simulink model "State_Flowc"  (R2017a)
settings: Solver=FixedStepDiscrete  StartTime=0.0  StopTime=inf  FixedStep=0.001  RelTol=1e-3  EnableMultiTasking=on
libraries: xpcethercatlib x31, simulink x4, simulink_extras x4, commutil2 x2
(part 1 of 2)
settings Model: xpc_rtwmakecfg_data=_xpcethercatlib_  SimulationMode=external  Creator=simoc  LastModifiedBy=Danie
settings SolverCC: EnableConcurrentExecution=on  ConcurrentTasks=on  AutoInsertRateTranBlk=on
settings DataIOCC: SaveFormat=StructureWithTime
settings OptimizationCC: BlockReduction=off  OptimizeBlockIOStorage=off  BufferReuse=off  GlobalBufferReuse=off  ExpressionFolding=off  LocalBlockOutputs=off
settings HardwareCC: ProdBitPerPointer=32  ProdBitPerSizeT=32  ProdBitPerPtrDiffT=32  ProdLargestAtomicFloat=None  ProdWordSize=32  ProdLongLongMode=on  ProdHWDeviceType=Generic->32-bit x86 compatible
settings RTWCC: SystemTargetFile=slrt.tlc  TemplateMakefile=slrt_default_tmf  Description=Simulink Real-Time  RTWCompilerOptimization=on
settings SimulinkRealTimeCC: xPCConcurrentTasks=on

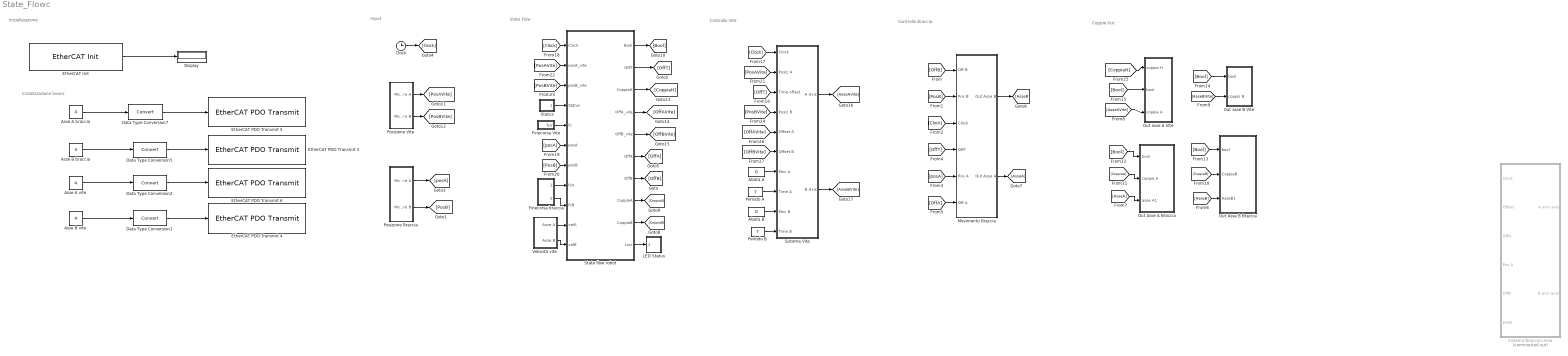
== system State_Flowc ==
  note: Input
  note: State Flow
  note: Coppie Out
  note: Controllo Braccia
  note: Controllo Vite
  note: Inizializzazione
  note: Inizializzazione lavoro
  Alzata A : Constant  Value=0
  "Alzata B " : Constant  Value=0
  Asse A braccia : Constant  Value=4
  Asse A vite : Constant  Value=4
  Asse B braccia : Constant  Value=4
  Asse B vite : Constant  Value=4
  Clock : Clock
  Data Type Conversion{1..2,5,7} (4 alike) : DataTypeConversion
  Display : Display
  "EtherCAT Init " : xpcethercatlib/EtherCAT Init   Priority=0  config_file=C:\Users\Danie\Downloads\final_net.xml  device_id=0  pci_bus=4  pci_slot=1  dctuning=0  enaDebug=off  enaDC=on  errLink=off  masterDbg=off  stateChgDbg=off  baseClock=off  masterCfg=off  logFile='c:\dbglog.txt'  sample_time=0.001000  DCMode=1
      settings: SourceProductName=Simulink Real-Time  SourceProductBaseCode=XP
  EtherCAT PDO Transmit 3 : xpcethercatlib/EtherCAT PDO Transmit   Priority=3  sig_name=AZ2.Receive PDO 1.Axis A Modes of operation  sig_offset=264  sig_type=int8  type_size=8  sig_dim=1  device_id=0  sample_time=0.001000
      settings: SourceProductName=Simulink Real-Time  SourceProductBaseCode=XP
  EtherCAT PDO Transmit 4 : xpcethercatlib/EtherCAT PDO Transmit   Priority=3  sig_name=AZ2.Receive PDO 1.Axis A Modes of operation  sig_offset=264  sig_type=int8  type_size=8  sig_dim=1  device_id=0  sample_time=0.001000
      settings: SourceProductName=Simulink Real-Time  SourceProductBaseCode=XP
  EtherCAT PDO Transmit 5 : xpcethercatlib/EtherCAT PDO Transmit   Priority=3  sig_name=AZ2.Receive PDO 2.Axis B Modes of operation  sig_offset=288  sig_type=int8  type_size=8  sig_dim=1  device_id=0  sample_time=0.001000
      settings: SourceProductName=Simulink Real-Time  SourceProductBaseCode=XP
  EtherCAT PDO Transmit 6 : xpcethercatlib/EtherCAT PDO Transmit   Priority=3  sig_name=AZ2.Receive PDO 1.Axis A Modes of operation  sig_offset=264  sig_type=int8  type_size=8  sig_dim=1  device_id=0  sample_time=0.001000
      settings: SourceProductName=Simulink Real-Time  SourceProductBaseCode=XP
  Finecorsa Vite : Subsystem
  Finecorsa braccia : Subsystem
  LED Status : Subsystem
  Movimento Braccia : Subsystem
  Out Asse A Braccia : Subsystem
  Out Asse B Braccia : Subsystem
  Out asse A Vite : Subsystem
  Out asse B Vite : Subsystem
  Periodo A : Constant  Value=7
  Periodo B : Constant  Value=7
  "Posizione Braccia " : Subsystem
  Posizione Vite : Subsystem
  Sistema Braccia Linea : Subsystem  Commented=on
  Sistema Vite : Subsystem
  State flow robot : Stateflow chart  TreatAsAtomicUnit=on
  Status : Subsystem
  "Velocita vite " : Subsystem
  wires:
  "EtherCAT Init "/1 -> Display/1
  Data Type Conversion7/1 -> EtherCAT PDO Transmit 5/1
  Asse A braccia/1 -> Data Type Conversion7/1
  Data Type Conversion5/1 -> EtherCAT PDO Transmit 3/1
  Asse B braccia/1 -> Data Type Conversion5/1
  Clock/1 -> [Clock]
  State flow robot/1(Bool) -> [Bool]
  Data Type Conversion1/1 -> EtherCAT PDO Transmit 4/1
  Asse B vite/1 -> Data Type Conversion1/1
  Data Type Conversion2/1 -> EtherCAT PDO Transmit 6/1
  Asse A vite/1 -> Data Type Conversion2/1
  Posizione Vite/2(Motore B) -> [PosBVite]
  Status/1(Word) -> State flow robot/4(Status)
  State flow robot/2(OffT) -> [OffT]
  Alzata A/1 -> Sistema Vite/7(Mov A)
  Periodo A/1 -> Sistema Vite/8(Time A)
  "Alzata B "/1 -> Sistema Vite/9(Mov B)
  Periodo B/1 -> Sistema Vite/10(Time B)
  Finecorsa Vite/1(fcV) -> State flow robot/5(fc)
  Finecorsa braccia/1(Asse A) -> State flow robot/8(fcA)
  Finecorsa braccia/2(Asse B) -> State flow robot/9(fcB)
  "Posizione Braccia "/2(Motore B) -> [PosB]
  "Posizione Braccia "/1(Motore A) -> [posA]
  Posizione Vite/1(Motore A) -> [PosAVite]
  State flow robot/10(Luci) -> LED Status/1(Luci)
  "Velocita vite "/1(Asse A) -> State flow robot/10(velA)
  "Velocita vite "/2(Asse B) -> State flow robot/11(velB)
  State flow robot/7(OffB) -> [OffB]
  State flow robot/6(OffA) -> [OffA]
  [AsseB] -> Out Asse B Braccia/3(AsseB1)
  [AsseA] -> Out Asse A Braccia/3(asse A1)
  [CoppiaB] -> Out Asse B Braccia/2(CoppiaB)
  State flow robot/9(CoppiaB) -> [CoppiaB]
  State flow robot/8(CoppiaA) -> [CoppiaA]
  [CoppiaA] -> Out Asse A Braccia/2(coppia A)
  [Bool] -> Out Asse A Braccia/1(bool)
  [Bool] -> Out Asse B Braccia/1(bool)
  [Bool] -> Out asse B Vite/1(bool)
  [Bool] -> Out asse A Vite/2(bool)
  [OffT] -> Sistema Vite/3(Time offset)
  [Clock] -> Sistema Vite/1(Clock)
  [Clock] -> State flow robot/1(Clock)
  [posA] -> State flow robot/6(posA)
  [PosB] -> State flow robot/7(posB)
  [PosAVite] -> Sistema Vite/2(Posiz A)
  [PosAVite] -> State flow robot/2(posA_vite)
  [PosBVite] -> State flow robot/3(posB_vite)
  [PosBVite] -> Sistema Vite/4(Posiz B)
  State flow robot/3(CoppiaH) -> [CoppiaH]
  [CoppiaH] -> Out asse A Vite/1(coppia H)
  State flow robot/4(OffA_vite) -> [OffAVite]
  [OffAVite] -> Sistema Vite/5(Offset A)
  State flow robot/5(OffB_vite) -> [OffBVite]
  [OffBVite] -> Sistema Vite/6(Offset B)
  [OffB] -> Movimento Braccia/1(Off B)
  [PosB] -> Movimento Braccia/2(Pos B)
  [Clock] -> Movimento Braccia/3(Clock)
  [OffT] -> Movimento Braccia/4(OffT)
  [posA] -> Movimento Braccia/5(Pos A)
  [OffA] -> Movimento Braccia/6(Off A)
  Movimento Braccia/1(Out Asse B) -> [AsseB]
  Movimento Braccia/2(Out Asse A) -> [AsseA]
  Sistema Vite/1(A Axis) -> [AsseAVite]
  [AsseAVite] -> Out asse A Vite/3(coppia A)
  Sistema Vite/2(B Axis) -> [AsseBVite]
  [AsseBVite] -> Out asse B Vite/2(coppis B)

== system State_Flowc/Finecorsa Vite ==
  Data Type Conversion8 : DataTypeConversion
  EtherCAT PDO Receive16 : xpcethercatlib/EtherCAT PDO Receive  Priority=2  sig_name=AZ2.Transmit PDO 3.General purpose inputs  sig_offset=440  sig_type=uint16  type_size=16  sig_dim=1  device_id=0  sample_time=0.001000
      settings: SourceProductName=Simulink Real-Time  SourceProductBaseCode=XP
  Integer to Bit Converter : commutil2/Integer to Bit Converter  nbits=16  signedInputValues=Unsigned  bitOrder=LSB first  outDtype=Inherit via internal rule
  Selector : Selector  InputPortWidth=16  IndexOptions=Index vector (dialog)  Indices=15  OutputSizes=1
  fcV : Outport
  wires:
  EtherCAT PDO Receive16/1 -> Data Type Conversion8/1
  Selector/1 -> fcV/1
  Data Type Conversion8/1 -> Integer to Bit Converter/1
  Integer to Bit Converter/1 -> Selector/1

== system State_Flowc/Finecorsa braccia ==
  Data Type Conversion8 : DataTypeConversion
  EtherCAT PDO Receive16 : xpcethercatlib/EtherCAT PDO Receive  Priority=2  sig_name=AZ1.Transmit PDO 3.General purpose inputs  sig_offset=184  sig_type=uint16  type_size=16  sig_dim=1  device_id=0  sample_time=0.001000
      settings: SourceProductName=Simulink Real-Time  SourceProductBaseCode=XP
  Integer to Bit Converter : commutil2/Integer to Bit Converter  nbits=16  signedInputValues=Unsigned  bitOrder=LSB first  outDtype=Inherit via internal rule
  Selector : Selector  InputPortWidth=16  IndexOptions=Index vector (dialog)  Indices=8  OutputSizes=1
  Selector1 : Selector  InputPortWidth=16  IndexOptions=Index vector (dialog)  Indices=15  OutputSizes=1
  Asse A : Outport
  Asse B : Outport  Port=2
  wires:
  Data Type Conversion8/1 -> Integer to Bit Converter/1
  Integer to Bit Converter/1 -> Selector1/1, Selector/1
  EtherCAT PDO Receive16/1 -> Data Type Conversion8/1
  Selector1/1 -> Asse B/1
  Selector/1 -> Asse A/1

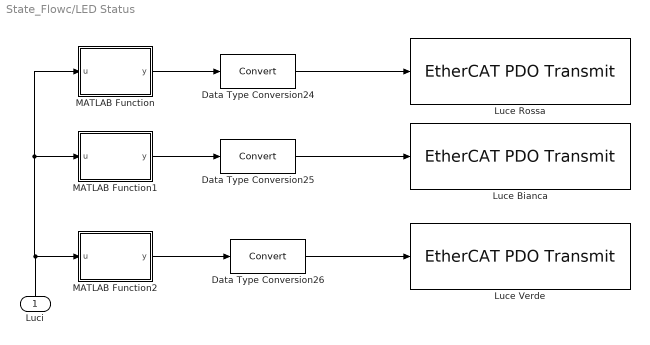
== system State_Flowc/LED Status ==
  Luci : Inport
  Data Type Conversion24 : DataTypeConversion
  Data Type Conversion25 : DataTypeConversion
  Data Type Conversion26 : DataTypeConversion
  Luce Bianca : xpcethercatlib/EtherCAT PDO Transmit   Priority=3  sig_name=Beckoff.Channel 6.Output  sig_offset=1  sig_type=boolean  type_size=1  sig_dim=1  device_id=0  sample_time=0.001000
      settings: SourceProductName=Simulink Real-Time  SourceProductBaseCode=XP
  "Luce Rossa " : xpcethercatlib/EtherCAT PDO Transmit   Priority=3  sig_name=Beckoff.Channel 8.Output  sig_offset=3  sig_type=boolean  type_size=1  sig_dim=1  device_id=0  sample_time=0.001000
      settings: SourceProductName=Simulink Real-Time  SourceProductBaseCode=XP
  Luce Verde : xpcethercatlib/EtherCAT PDO Transmit   Priority=3  sig_name=Beckoff.Channel 7.Output  sig_offset=2  sig_type=boolean  type_size=1  sig_dim=1  device_id=0  sample_time=0.001000
      settings: SourceProductName=Simulink Real-Time  SourceProductBaseCode=XP
  MATLAB Function : MATLAB Function  TreatAsAtomicUnit=on
  MATLAB Function1 : MATLAB Function  TreatAsAtomicUnit=on
  MATLAB Function2 : MATLAB Function  TreatAsAtomicUnit=on
  wires:
  MATLAB Function2/1(y) -> Data Type Conversion26/1
  MATLAB Function/1(y) -> Data Type Conversion24/1
  Data Type Conversion26/1 -> Luce Verde/1
  MATLAB Function1/1(y) -> Data Type Conversion25/1
  Data Type Conversion24/1 -> "Luce Rossa "/1
  Data Type Conversion25/1 -> Luce Bianca/1
  Luci/1 -> MATLAB Function/1(u), MATLAB Function1/1(u), MATLAB Function2/1(u)

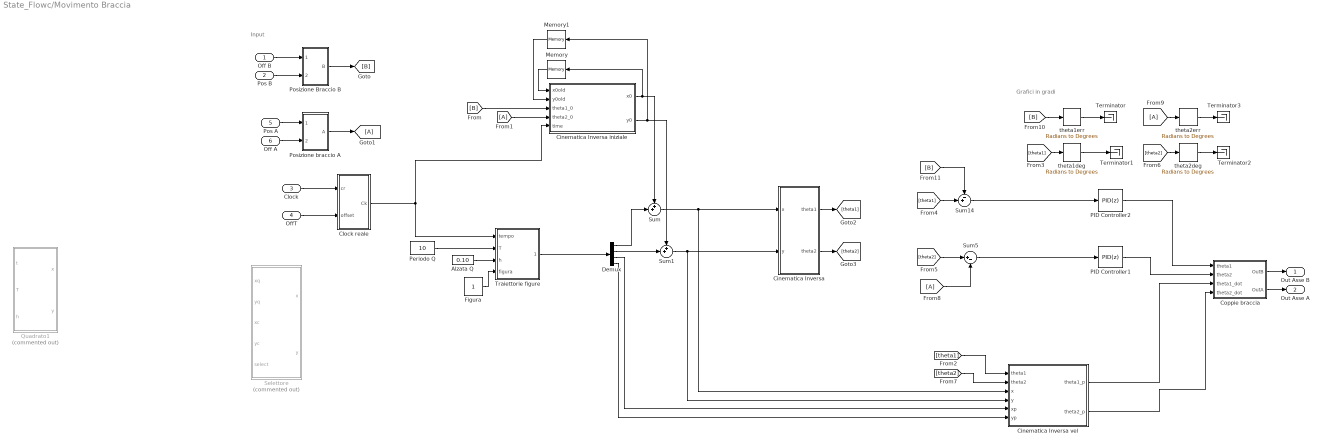
== system State_Flowc/Movimento Braccia ==
  note: Input
  note: Grafici in gradi
  Off B : Inport
  Pos B : Inport  Port=2
  Clock : Inport  Port=3
  OffT : Inport  Port=4
  Pos A : Inport  Port=5
  Off A : Inport  Port=6
  Alzata Q : Constant  Value=0.10
  Cinematica Inversa : MATLAB Function  TreatAsAtomicUnit=on
  Cinematica Inversa iniziale : MATLAB Function  TreatAsAtomicUnit=on
  Cinematica Inversa vel : MATLAB Function  TreatAsAtomicUnit=on
  Clock reale : Subsystem
  Coppie braccia : Subsystem
  Demux : Demux
  Figura : Constant
  Memory : Memory
  Memory1 : Memory
  PID Controller1 : simulink/Continuous/PID Controller  Controller=PID  TimeDomain=Discrete-time  SampleTime=-1  IntegratorMethod=Forward Euler  FilterMethod=Forward Euler  Form=Parallel  UseFilter=on  ControllerParametersSource=internal  P=3e+05  I=100  D=0  N=100  InitialConditionSource=internal  InitialConditionForIntegrator=0  InitialConditionForFilter=0  ExternalReset=none  LimitOutput=off  UpperSaturationLimit=inf  LowerSaturationLimit=-inf  LinearizeAsGain=on  AntiWindupMode=none  Kb=1  TrackingMode=off  Kt=1  PParamMin=[]  PParamMax=[]  IParamMin=[]  IParamMax=[]  DParamMin=[]  DParamMax=[]  NParamMin=[]  NParamMax=[]  KbParamMin=[]  KbParamMax=[]  KtParamMin=[]  KtParamMax=[]  POutMin=[]  POutMax=[]  IOutMin=[]  IOutMax=[]  DOutMin=[]  DOutMax=[]  NOutMin=[]  NOutMax=[]  KbOutMin=[]  KbOutMax=[]  KtOutMin=[]  KtOutMax=[]  IntegratorOutMin=[]  IntegratorOutMax=[]  FilterOutMin=[]  FilterOutMax=[]  SumOutMin=[]  SumOutMax=[]  SumI1OutMin=[]  SumI1OutMax=[]  SumI2OutMin=[]  SumI2OutMax=[]  SumI3OutMin=[]  SumI3OutMax=[]  SumDOutMin=[]  SumDOutMax=[]  SaturationOutMin=[]  SaturationOutMax=[]  IntegratorContinuousStateAttributes=''  IntegratorStateMustResolveToSignalObject=off  IntegratorRTWStateStorageClass=Auto  FilterContinuousStateAttributes=''  FilterStateMustResolveToSignalObject=off  FilterRTWStateStorageClass=Auto  DifferentiatorICPrevScaledInput=0  DifferentiatorOutMin=[]  DifferentiatorOutMax=[]  InitialConditionSetting=State (most efficient)
  PID Controller2 : simulink/Continuous/PID Controller  Controller=PID  TimeDomain=Discrete-time  SampleTime=-1  IntegratorMethod=Forward Euler  FilterMethod=Forward Euler  Form=Parallel  UseFilter=on  ControllerParametersSource=internal  P=3e+05  I=100  D=0  N=100  InitialConditionSource=internal  InitialConditionForIntegrator=0  InitialConditionForFilter=0  ExternalReset=none  LimitOutput=off  UpperSaturationLimit=inf  LowerSaturationLimit=-inf  LinearizeAsGain=on  AntiWindupMode=none  Kb=1  TrackingMode=off  Kt=1  PParamMin=[]  PParamMax=[]  IParamMin=[]  IParamMax=[]  DParamMin=[]  DParamMax=[]  NParamMin=[]  NParamMax=[]  KbParamMin=[]  KbParamMax=[]  KtParamMin=[]  KtParamMax=[]  POutMin=[]  POutMax=[]  IOutMin=[]  IOutMax=[]  DOutMin=[]  DOutMax=[]  NOutMin=[]  NOutMax=[]  KbOutMin=[]  KbOutMax=[]  KtOutMin=[]  KtOutMax=[]  IntegratorOutMin=[]  IntegratorOutMax=[]  FilterOutMin=[]  FilterOutMax=[]  SumOutMin=[]  SumOutMax=[]  SumI1OutMin=[]  SumI1OutMax=[]  SumI2OutMin=[]  SumI2OutMax=[]  SumI3OutMin=[]  SumI3OutMax=[]  SumDOutMin=[]  SumDOutMax=[]  SaturationOutMin=[]  SaturationOutMax=[]  IntegratorContinuousStateAttributes=''  IntegratorStateMustResolveToSignalObject=off  IntegratorRTWStateStorageClass=Auto  FilterContinuousStateAttributes=''  FilterStateMustResolveToSignalObject=off  FilterRTWStateStorageClass=Auto  DifferentiatorICPrevScaledInput=0  DifferentiatorOutMin=[]  DifferentiatorOutMax=[]  InitialConditionSetting=State (most efficient)
  Periodo Q : Constant  Value=10
  Posizione Braccio B : Subsystem
  Posizione braccio A : Subsystem
  Quadrato1 : MATLAB Function  Commented=on  TreatAsAtomicUnit=on
  Selettore : MATLAB Function  Commented=on  TreatAsAtomicUnit=on
  Sum : Sum  Inputs=++|
  Sum1 : Sum  Inputs=++|
  Sum14 : Sum  Inputs=-+|
  Sum5 : Sum  Inputs=|+-
  Terminator{,1..3} (4 alike) : Terminator
  Traiettorie figure : Subsystem
  theta1deg : simulink_extras/Transformations/Radians to Degrees
  theta1err : simulink_extras/Transformations/Radians to Degrees
  theta2deg : simulink_extras/Transformations/Radians to Degrees
  theta2err : simulink_extras/Transformations/Radians to Degrees
  Out Asse B : Outport
  Out Asse A : Outport  Port=2
  wires:
  Sum5/1 -> PID Controller1/1
  Cinematica Inversa iniziale/2(y0) -> Sum1/1, Memory1/1
  Sum/1 -> Cinematica Inversa vel/3(x), Cinematica Inversa/1(x)
  Sum1/1 -> Cinematica Inversa vel/4(y), Cinematica Inversa/2(y)
  Sum14/1 -> PID Controller2/1
  Clock/1 -> Clock reale/1(cr)
  OffT/1 -> Clock reale/2(offset)
  Clock reale/1(Ck) -> Cinematica Inversa iniziale/5(time), Traiettorie figure/1(tempo)
  Cinematica Inversa iniziale/1(x0) -> Sum/1, Memory/1
  Memory1/1 -> Cinematica Inversa iniziale/2(y0old)
  Memory/1 -> Cinematica Inversa iniziale/1(x0old)
  theta1deg/1 -> Terminator1/1
  theta1err/1 -> Terminator/1
  theta2deg/1 -> Terminator2/1
  theta2err/1 -> Terminator3/1
  Posizione Braccio B/1(B) -> [B]
  Off B/1 -> Posizione Braccio B/1(Off B)
  Pos B/1 -> Posizione Braccio B/2(Pos B)
  Posizione braccio A/1(A) -> [A]
  Pos A/1 -> Posizione braccio A/1(Pos A)
  Off A/1 -> Posizione braccio A/2(Off A)
  PID Controller2/1 -> Coppie braccia/1(theta1)
  PID Controller1/1 -> Coppie braccia/2(theta2)
  Cinematica Inversa vel/1(theta1_p) -> Coppie braccia/3(theta1_dot)
  Cinematica Inversa vel/2(theta2_p) -> Coppie braccia/4(theta2_dot)
  Coppie braccia/1(OutB) -> Out Asse B/1
  Coppie braccia/2(OutA) -> Out Asse A/1
  [B] -> Cinematica Inversa iniziale/3(theta1_0)
  [A] -> Cinematica Inversa iniziale/4(theta2_0)
  Demux/1 -> Sum/2
  Demux/2 -> Sum1/2
  Demux/3 -> Cinematica Inversa vel/5(xp)
  Demux/4 -> Cinematica Inversa vel/6(yp)
  Cinematica Inversa/1(theta1) -> [theta1]
  [theta1] -> Sum14/2
  [theta1] -> theta1deg/1
  [theta1] -> Cinematica Inversa vel/1(theta1)
  Cinematica Inversa/2(theta2) -> [theta2]
  [theta2] -> Sum5/1
  [theta2] -> theta2deg/1
  [theta2] -> Cinematica Inversa vel/2(theta2)
  [A] -> Sum5/2
  [A] -> theta2err/1
  [B] -> theta1err/1
  [B] -> Sum14/1
  Periodo Q/1 -> Traiettorie figure/2(T)
  Alzata Q/1 -> Traiettorie figure/3(h)
  Traiettorie figure/1(Parametri) -> Demux/1
  Figura/1 -> Traiettorie figure/4(figura)

== system State_Flowc/Out Asse A Braccia ==
  note: Invio motore asse A
  bool : Inport
  coppia A : Inport  Port=2
  asse A1 : Inport  Port=3
  Data Type Conversion3 : DataTypeConversion
  EtherCAT PDO Transmit 1 : xpcethercatlib/EtherCAT PDO Transmit   Priority=3  sig_name=AZ1.Receive PDO 1.Axis A Target Torque  sig_offset=16  sig_type=int16  type_size=16  sig_dim=1  device_id=0  sample_time=0.001000
      settings: SourceProductName=Simulink Real-Time  SourceProductBaseCode=XP
  Fungo : Subsystem
  Saturation : Saturate  UpperLimit=2500  LowerLimit=-2500
  Switch1 : Switch  Criteria=u2 > Threshold  Threshold=3
  wires:
  Data Type Conversion3/1 -> EtherCAT PDO Transmit 1/1
  bool/1 -> Switch1/2
  asse A1/1 -> Switch1/1
  coppia A/1 -> Switch1/3
  Switch1/1 -> Fungo/1(In1)
  Fungo/1(Out1) -> Saturation/1
  Saturation/1 -> Data Type Conversion3/1

== system State_Flowc/Out Asse B Braccia ==
  note: Invio motore Asse B
  bool : Inport
  CoppiaB : Inport  Port=2
  AsseB1 : Inport  Port=3
  Data Type Conversion4 : DataTypeConversion
  EtherCAT PDO Transmit 7 : xpcethercatlib/EtherCAT PDO Transmit   Priority=3  sig_name=AZ1.Receive PDO 2.Axis B Target Torque  sig_offset=40  sig_type=int16  type_size=16  sig_dim=1  device_id=0  sample_time=0.001000
      settings: SourceProductName=Simulink Real-Time  SourceProductBaseCode=XP
  Fungo : Subsystem
  Saturation : Saturate  UpperLimit=2500  LowerLimit=-2500
  Switch1 : Switch  Criteria=u2 > Threshold  Threshold=3
  wires:
  Data Type Conversion4/1 -> EtherCAT PDO Transmit 7/1
  AsseB1/1 -> Switch1/1
  Switch1/1 -> Fungo/1(In1)
  CoppiaB/1 -> Switch1/3
  bool/1 -> Switch1/2
  Fungo/1(Out1) -> Saturation/1
  Saturation/1 -> Data Type Conversion4/1

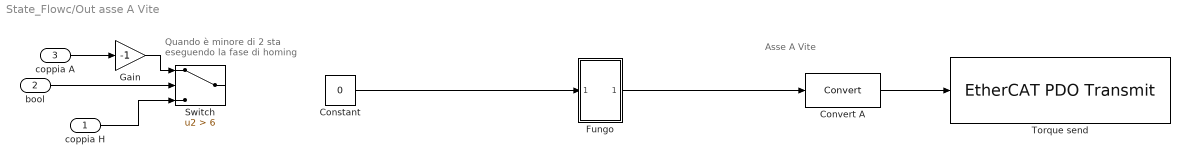
== system State_Flowc/Out asse A Vite ==
  note: Quando è minore di 2 sta
      |  eseguendo la fase di homing
  note: Asse A Vite
  coppia H : Inport
  bool : Inport  Port=2
  coppia A : Inport  Port=3
  Constant : Constant  Value=0
  Convert A : DataTypeConversion
  Fungo : Subsystem
  Gain : Gain  Gain=-1
  Switch : Switch  Criteria=u2 > Threshold  Threshold=6
  Torque send : xpcethercatlib/EtherCAT PDO Transmit   Priority=3  sig_name=AZ2.Receive PDO 1.Axis A Target Torque  sig_offset=272  sig_type=int16  type_size=16  sig_dim=1  device_id=0  sample_time=0.001000
      settings: SourceProductName=Simulink Real-Time  SourceProductBaseCode=XP
  wires:
  bool/1 -> Switch/2
  Convert A/1 -> Torque send/1
  coppia H/1 -> Switch/3
  coppia A/1 -> Gain/1
  Gain/1 -> Switch/1
  Fungo/1(Out1) -> Convert A/1
  Constant/1 -> Fungo/1(In1)

== system State_Flowc/Out asse B Vite ==
  note: Asse B Vite
  bool : Inport
  coppis B : Inport  Port=2
  Constant1 : Constant  Value=0
  Convert B : DataTypeConversion
  EtherCAT PDO Transmit 2 : xpcethercatlib/EtherCAT PDO Transmit   Priority=3  sig_name=AZ2.Receive PDO 2.Axis B Target Torque  sig_offset=296  sig_type=int16  type_size=16  sig_dim=1  device_id=0  sample_time=0.001000
      settings: SourceProductName=Simulink Real-Time  SourceProductBaseCode=XP
  Fungo : Subsystem
  Switch2 : Switch  Criteria=u2 > Threshold  Threshold=6
  wires:
  bool/1 -> Switch2/2
  coppis B/1 -> Switch2/1
  Constant1/1 -> Switch2/3
  Convert B/1 -> EtherCAT PDO Transmit 2/1
  Switch2/1 -> Fungo/1(In1)
  Fungo/1(Out1) -> Convert B/1

== system State_Flowc/Posizione Braccia  ==
  Motore braccia A : xpcethercatlib/EtherCAT PDO Receive  Priority=2  sig_name=AZ1.Transmit PDO 1.Axis A Actual motor position  sig_offset=16  sig_type=int32  type_size=32  sig_dim=1  device_id=0  sample_time=0.001000
      settings: SourceProductName=Simulink Real-Time  SourceProductBaseCode=XP
  Motore braccia B : xpcethercatlib/EtherCAT PDO Receive  Priority=2  sig_name=AZ1.Transmit PDO 2.Axis B Actual motor position  sig_offset=104  sig_type=int32  type_size=32  sig_dim=1  device_id=0  sample_time=0.001000
      settings: SourceProductName=Simulink Real-Time  SourceProductBaseCode=XP
  convert : DataTypeConversion
  "convert 10 " : DataTypeConversion
  Motore A : Outport
  Motore B : Outport  Port=2
  wires:
  Motore braccia B/1 -> "convert 10 "/1
  Motore braccia A/1 -> convert/1
  "convert 10 "/1 -> Motore B/1
  convert/1 -> Motore A/1

== system State_Flowc/Posizione Vite ==
  Motore vite A : xpcethercatlib/EtherCAT PDO Receive  Priority=2  sig_name=AZ2.Transmit PDO 1.Axis A Actual motor position  sig_offset=272  sig_type=int32  type_size=32  sig_dim=1  device_id=0  sample_time=0.001000
      settings: SourceProductName=Simulink Real-Time  SourceProductBaseCode=XP
  Motore vite B : xpcethercatlib/EtherCAT PDO Receive  Priority=2  sig_name=AZ2.Transmit PDO 2.Axis B Actual motor position  sig_offset=360  sig_type=int32  type_size=32  sig_dim=1  device_id=0  sample_time=0.001000
      settings: SourceProductName=Simulink Real-Time  SourceProductBaseCode=XP
  convert : DataTypeConversion
  "convert 10 " : DataTypeConversion
  Motore A : Outport
  Motore B : Outport  Port=2
  wires:
  Motore vite B/1 -> "convert 10 "/1
  Motore vite A/1 -> convert/1
  "convert 10 "/1 -> Motore B/1
  convert/1 -> Motore A/1

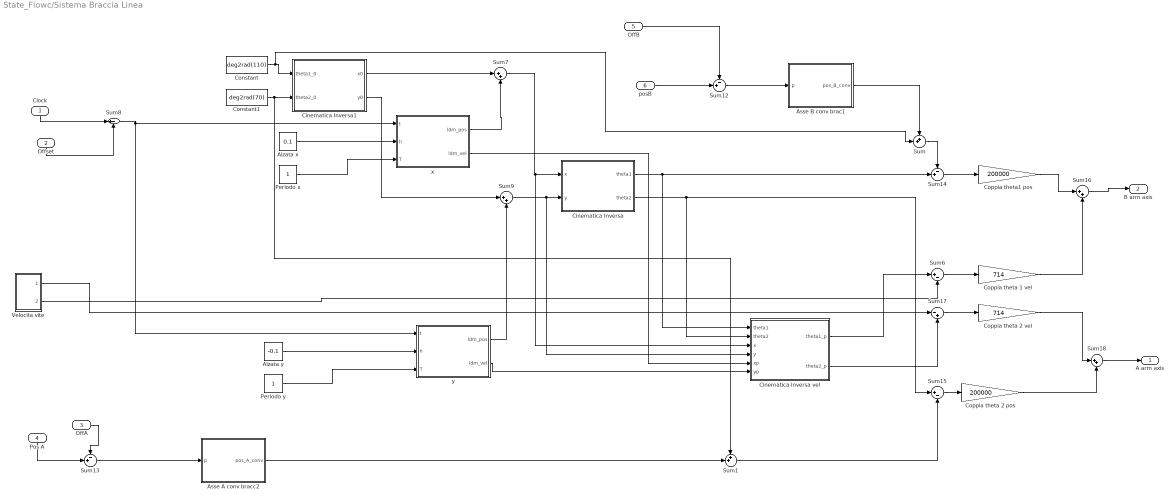
== system State_Flowc/Sistema Braccia Linea ==
  Clock : Inport
  Offset : Inport  Port=2
  OffA : Inport  Port=3
  Pos A : Inport  Port=4
  OffB : Inport  Port=5
  posB : Inport  Port=6
  Alzata x : Constant  Value=0.1
  Alzata y : Constant  Value=-0.1
  Asse A conv bracc2 : MATLAB Function  TreatAsAtomicUnit=on
  Asse B conv brac1 : MATLAB Function  TreatAsAtomicUnit=on
  Cinematica Inversa : MATLAB Function  TreatAsAtomicUnit=on
  Cinematica Inversa vel : MATLAB Function  TreatAsAtomicUnit=on
  Cinematica Inversa1 : MATLAB Function  TreatAsAtomicUnit=on
  Constant : Constant  Value=deg2rad(110)
  Constant1 : Constant  Value=deg2rad(70)
  Coppia theta 1 vel : Gain  Gain=714
  Coppia theta 2 pos : Gain  Gain=200000
  Coppia theta 2 vel : Gain  Gain=714
  Coppia theta1 pos : Gain  Gain=200000
  Periodo x : Constant
  Periodo y : Constant
  Sum : Sum  Inputs=++|
  Sum1 : Sum  Inputs=++|
  Sum12 : Sum  Inputs=-+|
  Sum13 : Sum  Inputs=-+|
  Sum14 : Sum  Inputs=-+|
  Sum15 : Sum  Inputs=|+-
  Sum{7,9,16,18} (4 alike) : Sum  Inputs=|++
  Sum17 : Sum  Inputs=|-+
  Sum6 : Sum  Inputs=|+-
  Sum8 : Sum  Inputs=|+-
  "Velocita vite " : Subsystem
  x : MATLAB Function  TreatAsAtomicUnit=on
  y : MATLAB Function  TreatAsAtomicUnit=on
  "A arm axis " : Outport
  B arm axis : Outport  Port=2
  wires:
  Sum15/1 -> Coppia theta 2 pos/1
  OffB/1 -> Sum12/1
  x/1(ldm_pos) -> Sum7/2
  posB/1 -> Sum12/2
  y/2(ldm_vel) -> Cinematica Inversa vel/6(yp)
  Cinematica Inversa/2(theta2) -> Cinematica Inversa vel/2(theta2), Sum15/1
  Cinematica Inversa1/2(y0) -> Sum9/1
  Constant1/1 -> Sum1/1, Cinematica Inversa1/2(theta2_0)
  y/1(ldm_pos) -> Sum9/2
  Sum12/1 -> Asse B conv brac1/1(p)
  Clock/1 -> Sum8/1
  Alzata x/1 -> x/2(h)
  Sum7/1 -> Cinematica Inversa vel/3(x), Cinematica Inversa/1(x)
  Constant/1 -> Sum/2, Cinematica Inversa1/1(theta1_0)
  Cinematica Inversa1/1(x0) -> Sum7/1
  Alzata y/1 -> y/2(h)
  Sum6/1 -> Coppia theta 1 vel/1
  Pos A/1 -> Sum13/2
  x/2(ldm_vel) -> Cinematica Inversa vel/5(xp)
  Sum8/1 -> y/1(t), x/1(t)
  Periodo x/1 -> x/3(T)
  Cinematica Inversa vel/2(theta2_p) -> Sum17/2
  Offset/1 -> Sum8/2
  Periodo y/1 -> y/3(T)
  Coppia theta 2 pos/1 -> Sum18/2
  "Velocita vite "/2(Asse B) -> Sum6/2
  Cinematica Inversa vel/1(theta1_p) -> Sum6/1
  OffA/1 -> Sum13/1
  Sum9/1 -> Cinematica Inversa vel/4(y), Cinematica Inversa/2(y)
  Coppia theta1 pos/1 -> Sum16/1
  Cinematica Inversa/1(theta1) -> Sum14/2, Cinematica Inversa vel/1(theta1)
  Sum13/1 -> Asse A conv bracc2/1(p)
  Coppia theta 1 vel/1 -> Sum16/2
  Coppia theta 2 vel/1 -> Sum18/1
  Sum14/1 -> Coppia theta1 pos/1
  Sum17/1 -> Coppia theta 2 vel/1
  Asse B conv brac1/1(pos_B_conv) -> Sum/1
  "Velocita vite "/1(Asse A) -> Sum17/1
  Sum16/1 -> B arm axis/1
  Sum18/1 -> "A arm axis "/1
  Asse A conv bracc2/1(pos_A_conv) -> Sum1/2
  Sum/1 -> Sum14/1
  Sum1/1 -> Sum15/2

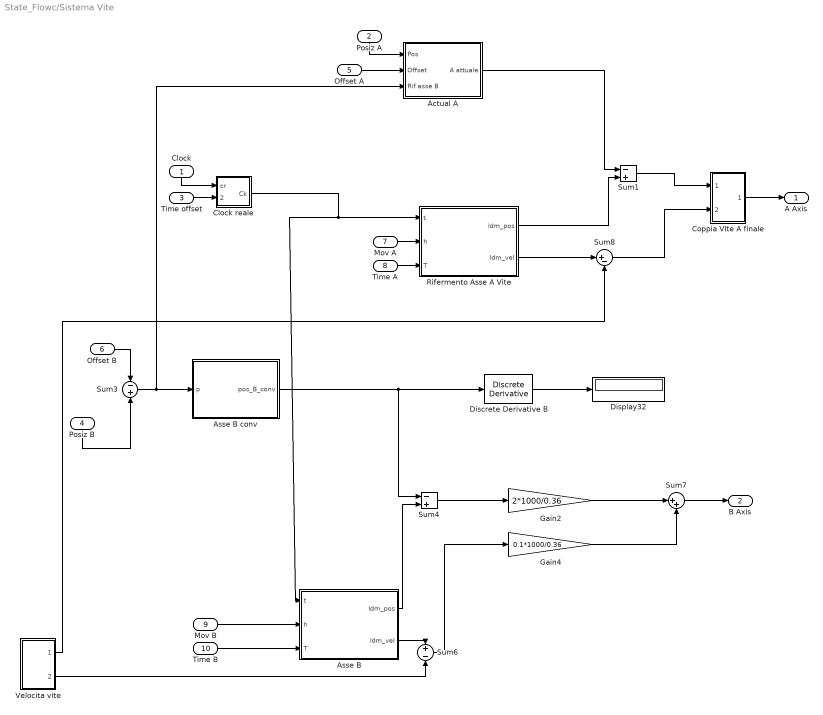
== system State_Flowc/Sistema Vite ==
  Clock : Inport
  Posiz A : Inport  Port=2
  Time offset : Inport  Port=3
  Posiz B : Inport  Port=4
  Offset A : Inport  Port=5
  Offset B : Inport  Port=6
  Mov A : Inport  Port=7
  Time A : Inport  Port=8
  Mov B : Inport  Port=9
  Time B : Inport  Port=10
  Actual A : Subsystem
  Asse B : MATLAB Function  TreatAsAtomicUnit=on
  Asse B conv : MATLAB Function  TreatAsAtomicUnit=on
  Clock reale : Subsystem
  Coppia VIte A finale : Subsystem
  Discrete Derivative B : simulink/Discrete/Discrete Derivative  gainval=1.0  ICPrevScaledInput=0.0  OutMin=[]  OutMax=[]  OutDataType=fixdt(1, 16)  OutScaling=2^-10  DoSatur=off
  Display32 : Display
  Gain2 : Gain  Gain=2*1000/0.36
  Gain4 : Gain  Gain=0.1*1000/0.36
  Rifermento Asse A Vite : MATLAB Function  TreatAsAtomicUnit=on
  Sum1 : Sum  Inputs=-+
  Sum3 : Sum  Inputs=-|+
  Sum4 : Sum  Inputs=-+
  Sum6 : Sum  Inputs=+|-
  Sum7 : Sum  Inputs=|++
  Sum8 : Sum  Inputs=|+-
  "Velocita vite " : Subsystem
  A Axis : Outport
  B Axis : Outport  Port=2
  wires:
  Clock/1 -> Clock reale/1(cr)
  Posiz A/1 -> Actual A/1(Pos)
  Offset A/1 -> Actual A/2(Offset)
  Coppia VIte A finale/1(Coppia) -> A Axis/1
  Sum7/1 -> B Axis/1
  Mov A/1 -> Rifermento Asse A Vite/2(h)
  Time A/1 -> Rifermento Asse A Vite/3(T)
  "Velocita vite "/2(Asse B) -> Sum6/2
  Offset B/1 -> Sum3/1
  Asse B conv/1(pos_B_conv) -> Discrete Derivative B/1, Sum4/1
  Asse B/1(ldm_pos) -> Sum4/2
  Sum4/1 -> Gain2/1
  Sum3/1 -> Actual A/3(Rif asse B), Asse B conv/1(p)
  Gain4/1 -> Sum7/2
  Rifermento Asse A Vite/1(ldm_pos) -> Sum1/2
  Mov B/1 -> Asse B/2(h)
  Asse B/2(ldm_vel) -> Sum6/1
  "Velocita vite "/1(Asse A) -> Sum8/2
  Gain2/1 -> Sum7/1
  Sum6/1 -> Gain4/1
  Time B/1 -> Asse B/3(T)
  Rifermento Asse A Vite/2(ldm_vel) -> Sum8/1
  Sum1/1 -> Coppia VIte A finale/1(Pos)
  Sum8/1 -> Coppia VIte A finale/2(Vel)
  Actual A/1(A attuale) -> Sum1/1
  Clock reale/1(Ck) -> Asse B/1(t), Rifermento Asse A Vite/1(t)
  Time offset/1 -> Clock reale/2(offset)
  Discrete Derivative B/1 -> Display32/1
  Posiz B/1 -> Sum3/2

== system State_Flowc/State flow robot/Homing ==
  fc : Inport  OutDataTypeStr=double  PortDimensions=1
  fcA : Inport  Port=2  OutDataTypeStr=double  PortDimensions=1
  fcB : Inport  Port=3  OutDataTypeStr=double  PortDimensions=1
  f : TriggerPort  TriggerType=function-call  VariantControl=Variant  SampleTimeType=periodic  SampleTime=-1
      settings: CopyFcn=Stateflow.SLINSF.SimulinkMan.removeBlockPreDeleteFcn  PreDeleteFcn=Stateflow.SLINSF.SimulinkMan.unsafePredeleteFcn
  MATLAB Function : MATLAB Function  TreatAsAtomicUnit=on
  CA : Outport
  CB : Outport  Port=2
  CH : Outport  Port=3
  wires:
  fc/1 -> MATLAB Function/1(fc)
  fcB/1 -> MATLAB Function/3(fcB)
  fcA/1 -> MATLAB Function/2(fcA)
  MATLAB Function/1(CA) -> CA/1
  MATLAB Function/2(CB) -> CB/1
  MATLAB Function/3(CH) -> CH/1

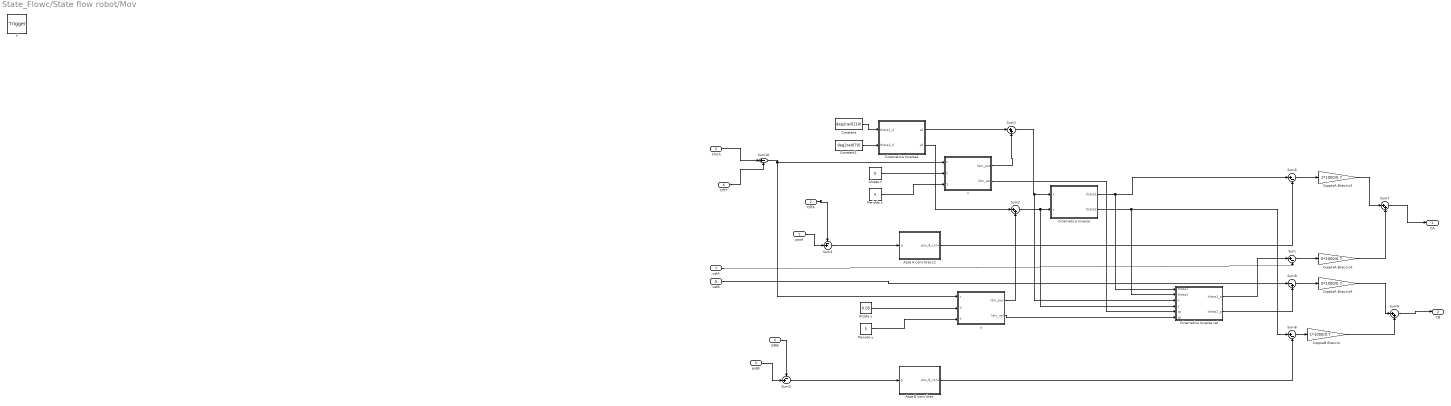
== system State_Flowc/State flow robot/Mov ==
  posA : Inport  OutDataTypeStr=double  PortDimensions=1
  OffA : Inport  Port=2  OutDataTypeStr=double  PortDimensions=1
  posB : Inport  Port=3  OutDataTypeStr=double  PortDimensions=1
  OffB : Inport  Port=4  OutDataTypeStr=double  PortDimensions=1
  Clock : Inport  Port=5  OutDataTypeStr=double  PortDimensions=1
  OffT : Inport  Port=6  OutDataTypeStr=double  PortDimensions=1
  velA : Inport  Port=7  OutDataTypeStr=double  PortDimensions=1
  velB : Inport  Port=8  OutDataTypeStr=double  PortDimensions=1
  f : TriggerPort  TriggerType=function-call  VariantControl=Variant  SampleTimeType=periodic  SampleTime=-1
      settings: CopyFcn=Stateflow.SLINSF.SimulinkMan.removeBlockPreDeleteFcn  PreDeleteFcn=Stateflow.SLINSF.SimulinkMan.unsafePredeleteFcn
  Alzata x : Constant  Value=0
  Alzata y : Constant  Value=0.05
  Asse A conv bracc2 : MATLAB Function  TreatAsAtomicUnit=on
  Asse B conv brac : MATLAB Function  TreatAsAtomicUnit=on
  Cinematica Inversa : MATLAB Function  TreatAsAtomicUnit=on
  Cinematica Inversa vel : MATLAB Function  TreatAsAtomicUnit=on
  Cinematica Inversa1 : MATLAB Function  TreatAsAtomicUnit=on
  Constant : Constant  Value=deg2rad(110)
  Constant1 : Constant  Value=deg2rad(70)
  CoppiaA Braccio2 : Gain  Gain=1*1000/0.7
  CoppiaA Braccio3 : Gain  Gain=0*1000/0.7
  CoppiaA Braccio4 : Gain  Gain=0*1000/0.7
  CoppiaB Braccio : Gain  Gain=1*1000/0.7
  Periodo x : Constant  Value=5
  Periodo y : Constant  Value=5
  Sum{,5..6,10} (4 alike) : Sum  Inputs=|+-
  Sum{1..2,7,9} (4 alike) : Sum  Inputs=|++
  Sum3 : Sum  Inputs=-+|
  Sum4 : Sum  Inputs=-+|
  Sum8 : Sum  Inputs=|-+
  x : MATLAB Function  TreatAsAtomicUnit=on
  y : MATLAB Function  TreatAsAtomicUnit=on
  CA : Outport
  CB : Outport  Port=2
  wires:
  Sum7/1 -> CA/1
  CoppiaA Braccio4/1 -> Sum9/1
  CoppiaB Braccio/1 -> Sum9/2
  CoppiaA Braccio3/1 -> Sum7/2
  velB/1 -> Sum8/1
  Sum/1 -> CoppiaA Braccio3/1
  velA/1 -> Sum/2
  Sum8/1 -> CoppiaA Braccio4/1
  OffB/1 -> Sum3/1
  OffA/1 -> Sum4/1
  OffT/1 -> Sum10/2
  Asse A conv bracc2/1(pos_A_conv) -> Sum5/2
  posB/1 -> Sum3/2
  Alzata x/1 -> x/2(h)
  Clock/1 -> Sum10/1
  Sum6/1 -> CoppiaB Braccio/1
  Sum3/1 -> Asse B conv brac/1(p)
  Sum10/1 -> y/1(t), x/1(t)
  Sum4/1 -> Asse A conv bracc2/1(p)
  CoppiaA Braccio2/1 -> Sum7/1
  Sum5/1 -> CoppiaA Braccio2/1
  Sum9/1 -> CB/1
  Asse B conv brac/1(pos_B_conv) -> Sum6/2
  Periodo x/1 -> x/3(T)
  posA/1 -> Sum4/2
  Alzata y/1 -> y/2(h)
  Periodo y/1 -> y/3(T)
  x/1(ldm_pos) -> Sum1/2
  x/2(ldm_vel) -> Cinematica Inversa vel/5(xp)
  y/2(ldm_vel) -> Cinematica Inversa vel/6(yp)
  Cinematica Inversa/1(theta1) -> Cinematica Inversa vel/1(theta1), Sum5/1
  Cinematica Inversa/2(theta2) -> Cinematica Inversa vel/2(theta2), Sum6/1
  Cinematica Inversa vel/1(theta1_p) -> Sum/1
  Cinematica Inversa vel/2(theta2_p) -> Sum8/2
  Constant/1 -> Cinematica Inversa1/1(theta1_0)
  Constant1/1 -> Cinematica Inversa1/2(theta2_0)
  Cinematica Inversa1/1(x0) -> Sum1/1
  Sum1/1 -> Cinematica Inversa vel/3(x), Cinematica Inversa/1(x)
  Cinematica Inversa1/2(y0) -> Sum2/1
  y/1(ldm_pos) -> Sum2/2
  Sum2/1 -> Cinematica Inversa vel/4(y), Cinematica Inversa/2(y)

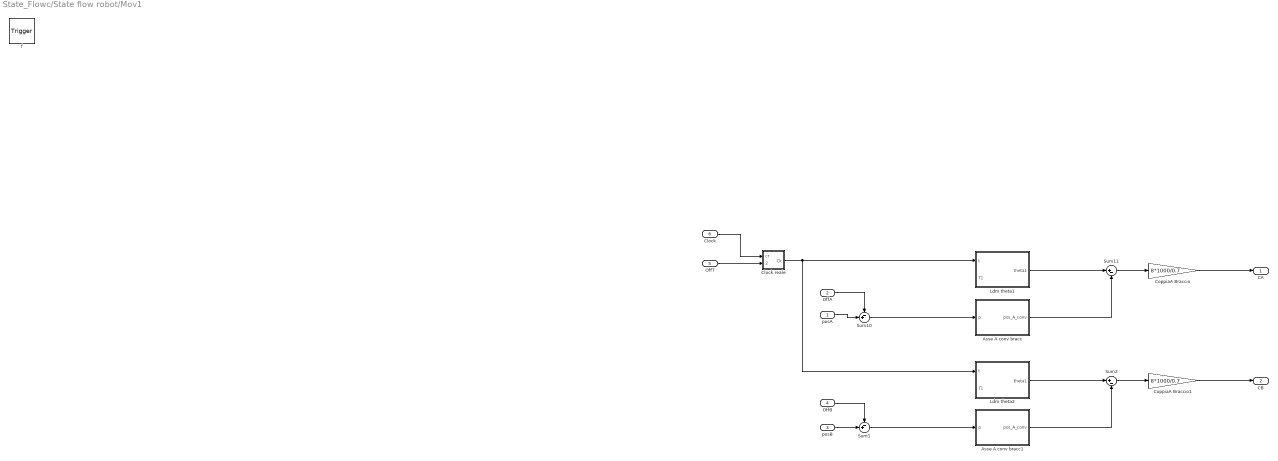
== system State_Flowc/State flow robot/Mov1 ==
  posA : Inport  OutDataTypeStr=double  PortDimensions=1
  OffA : Inport  Port=2  OutDataTypeStr=double  PortDimensions=1
  posB : Inport  Port=3  OutDataTypeStr=double  PortDimensions=1
  OffB : Inport  Port=4  OutDataTypeStr=double  PortDimensions=1
  OffT : Inport  Port=5  OutDataTypeStr=double  PortDimensions=1
  Clock : Inport  Port=6  OutDataTypeStr=double  PortDimensions=1
  f : TriggerPort  TriggerType=function-call  VariantControl=Variant  SampleTimeType=periodic  SampleTime=-1
      settings: CopyFcn=Stateflow.SLINSF.SimulinkMan.removeBlockPreDeleteFcn  PreDeleteFcn=Stateflow.SLINSF.SimulinkMan.unsafePredeleteFcn
  Asse A conv bracc : MATLAB Function  TreatAsAtomicUnit=on
  Asse A conv bracc1 : MATLAB Function  TreatAsAtomicUnit=on
  Clock reale : Subsystem
  CoppiaA Braccio : Gain  Gain=8*1000/0.7
  CoppiaA Braccio1 : Gain  Gain=8*1000/0.7
  Ldm theta1 : MATLAB Function  TreatAsAtomicUnit=on
  Ldm theta2 : MATLAB Function  TreatAsAtomicUnit=on
  Sum1 : Sum  Inputs=-+|
  Sum10 : Sum  Inputs=-+|
  Sum11 : Sum  Inputs=|+-
  Sum2 : Sum  Inputs=|+-
  CA : Outport
  CB : Outport  Port=2
  wires:
  CoppiaA Braccio/1 -> CA/1
  OffA/1 -> Sum10/1
  OffT/1 -> Clock reale/2(offset)
  Asse A conv bracc/1(pos_A_conv) -> Sum11/2
  Clock/1 -> Clock reale/1(cr)
  Ldm theta1/1(theta1) -> Sum11/1
  posA/1 -> Sum10/2
  Sum10/1 -> Asse A conv bracc/1(p)
  Sum11/1 -> CoppiaA Braccio/1
  OffB/1 -> Sum1/1
  posB/1 -> Sum1/2
  Ldm theta2/1(theta1) -> Sum2/1
  ? -> Ldm theta2/2(T1)
  CoppiaA Braccio1/1 -> CB/1
  Asse A conv bracc1/1(pos_A_conv) -> Sum2/2
  Sum1/1 -> Asse A conv bracc1/1(p)
  Clock reale/1(Ck) -> Ldm theta2/1(t), Ldm theta1/1(t)
  Sum2/1 -> CoppiaA Braccio1/1

== system State_Flowc/Status ==
  Data Type Conversion6 : DataTypeConversion
  Status Word : xpcethercatlib/EtherCAT PDO Receive  Priority=2  sig_name=AZ2.Transmit PDO 4.Axis A Status word  sig_offset=456  sig_type=uint16  type_size=16  sig_dim=1  device_id=0  sample_time=0.001000
      settings: SourceProductName=Simulink Real-Time  SourceProductBaseCode=XP
  Word : Outport
  wires:
  Data Type Conversion6/1 -> Word/1
  Status Word/1 -> Data Type Conversion6/1

== system State_Flowc/Velocita vite  ==
  EtherCAT PDO Receive14 : xpcethercatlib/EtherCAT PDO Receive  Priority=2  sig_name=AZ1.Transmit PDO 1.Axis A Actual motor velocity  sig_offset=48  sig_type=int32  type_size=32  sig_dim=1  device_id=0  sample_time=0.001000
      settings: SourceProductName=Simulink Real-Time  SourceProductBaseCode=XP
  EtherCAT PDO Receive15 : xpcethercatlib/EtherCAT PDO Receive  Priority=2  sig_name=AZ1.Transmit PDO 2.Axis B Actual motor velocity  sig_offset=136  sig_type=int32  type_size=32  sig_dim=1  device_id=0  sample_time=0.001000
      settings: SourceProductName=Simulink Real-Time  SourceProductBaseCode=XP
  Vel Asse A conv : MATLAB Function  TreatAsAtomicUnit=on
  Vel Asse B conv : MATLAB Function  TreatAsAtomicUnit=on
  Velocity A : DataTypeConversion
  Velocity B : DataTypeConversion
  Asse A : Outport
  Asse B : Outport  Port=2
  wires:
  EtherCAT PDO Receive15/1 -> Velocity B/1
  EtherCAT PDO Receive14/1 -> Velocity A/1
  Vel Asse A conv/1(vel_A_conv) -> Asse A/1
  Velocity B/1 -> Vel Asse B conv/1(p)
  Vel Asse B conv/1(vel_B_conv) -> Asse B/1
  Velocity A/1 -> Vel Asse A conv/1(vA)

== system State_Flowc/Movimento Braccia/Clock reale ==
  cr : Inport
  offset : Inport  Port=2
  Sum2 : Sum  Inputs=-+|
  Ck : Outport
  wires:
  Sum2/1 -> Ck/1
  offset/1 -> Sum2/1
  cr/1 -> Sum2/2

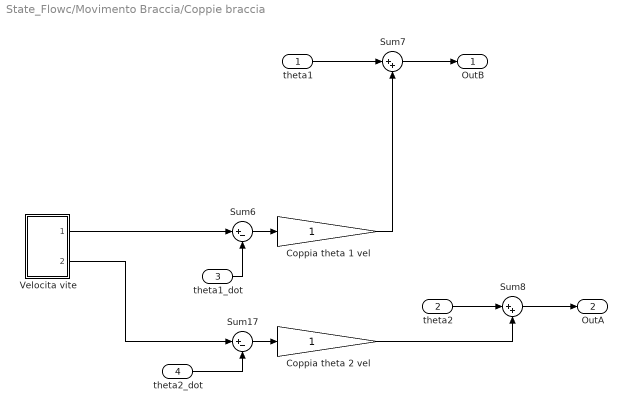
== system State_Flowc/Movimento Braccia/Coppie braccia ==
  theta1 : Inport
  theta2 : Inport  Port=2
  theta1_dot : Inport  Port=3
  theta2_dot : Inport  Port=4
  Coppia theta 1 vel : Gain
  Coppia theta 2 vel : Gain
  Sum17 : Sum  Inputs=|+-
  Sum6 : Sum  Inputs=|+-
  Sum7 : Sum  Inputs=|++
  Sum8 : Sum  Inputs=|++
  "Velocita vite " : Subsystem
  OutB : Outport
  OutA : Outport  Port=2
  wires:
  "Velocita vite "/1(Asse B) -> Sum6/1
  theta2_dot/1 -> Sum17/2
  Sum17/1 -> Coppia theta 2 vel/1
  theta2/1 -> Sum8/1
  theta1_dot/1 -> Sum6/2
  Sum7/1 -> OutB/1
  Coppia theta 2 vel/1 -> Sum8/2
  Sum6/1 -> Coppia theta 1 vel/1
  theta1/1 -> Sum7/1
  Sum8/1 -> OutA/1
  Coppia theta 1 vel/1 -> Sum7/2
  "Velocita vite "/2(Asse A) -> Sum17/1

== system State_Flowc/Movimento Braccia/Posizione Braccio B ==
  Off B : Inport
  Pos B : Inport  Port=2
  Asse B conv brac1 : MATLAB Function  TreatAsAtomicUnit=on
  Constant : Constant  Value=deg2rad(110)
  Sum12 : Sum  Inputs=-+|
  Sum2 : Sum  Inputs=++|
  B : Outport
  wires:
  Asse B conv brac1/1(pos_B_conv) -> Sum2/1
  Sum12/1 -> Asse B conv brac1/1(p)
  Pos B/1 -> Sum12/2
  Constant/1 -> Sum2/2
  Off B/1 -> Sum12/1
  Sum2/1 -> B/1

== system State_Flowc/Movimento Braccia/Posizione braccio A ==
  Pos A : Inport
  Off A : Inport  Port=2
  Asse A conv brac : MATLAB Function  TreatAsAtomicUnit=on
  Constant1 : Constant  Value=deg2rad(70)
  Sum3 : Sum  Inputs=++|
  Sum4 : Sum  Inputs=-+|
  A : Outport
  wires:
  Sum3/1 -> A/1
  Off A/1 -> Sum4/1
  Asse A conv brac/1(pos_A_conv) -> Sum3/2
  Constant1/1 -> Sum3/1
  Pos A/1 -> Sum4/2
  Sum4/1 -> Asse A conv brac/1(p)

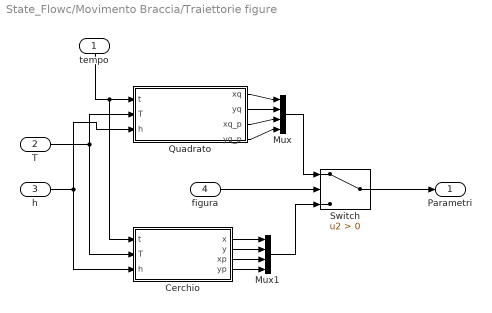
== system State_Flowc/Movimento Braccia/Traiettorie figure ==
  tempo : Inport
  T : Inport  Port=2
  h : Inport  Port=3
  figura : Inport  Port=4
  Cerchio : MATLAB Function  TreatAsAtomicUnit=on
  Mux : Mux
  Mux1 : Mux
  Quadrato : MATLAB Function  TreatAsAtomicUnit=on
  Switch : Switch  Criteria=u2 > Threshold
  Parametri : Outport
  wires:
  Mux1/1 -> Switch/3
  Switch/1 -> Parametri/1
  tempo/1 -> Cerchio/1(t), Quadrato/1(t)
  Quadrato/1(xq) -> Mux/1
  Quadrato/3(xq_p) -> Mux/3
  Quadrato/4(yq_p) -> Mux/4
  Quadrato/2(yq) -> Mux/2
  Cerchio/3(xp) -> Mux1/3
  Cerchio/4(yp) -> Mux1/4
  T/1 -> Quadrato/2(T), Cerchio/2(T)
  figura/1 -> Switch/2
  h/1 -> Quadrato/3(h), Cerchio/3(h)
  Mux/1 -> Switch/1
  Cerchio/1(x) -> Mux1/1
  Cerchio/2(y) -> Mux1/2

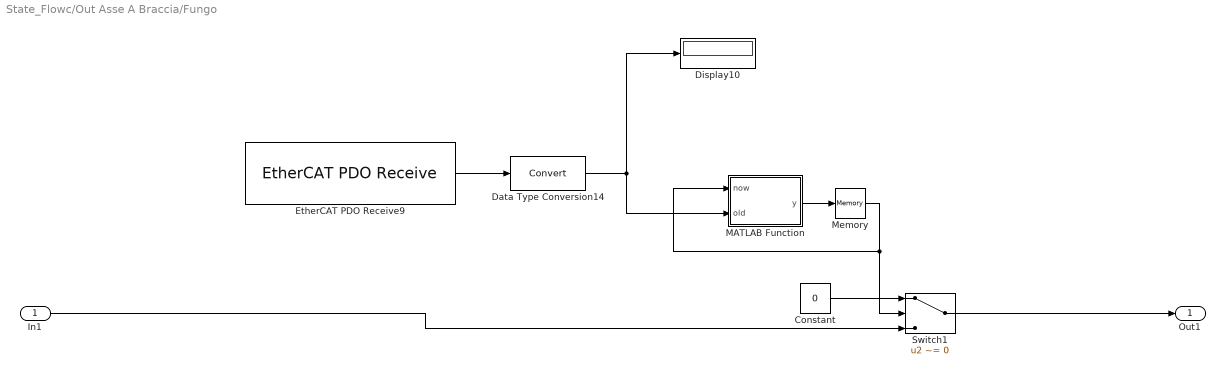
== system State_Flowc/Out Asse A Braccia/Fungo ==
  In1 : Inport
  Constant : Constant  Value=0
  Data Type Conversion14 : DataTypeConversion
  Display10 : Display
  EtherCAT PDO Receive9 : xpcethercatlib/EtherCAT PDO Receive  Priority=2  sig_name=Beckoff.Channel 1.Input  sig_offset=0  sig_type=boolean  type_size=1  sig_dim=1  device_id=0  sample_time=0.001000
      settings: SourceProductName=Simulink Real-Time  SourceProductBaseCode=XP
  MATLAB Function : MATLAB Function  TreatAsAtomicUnit=on
  Memory : Memory
  Switch1 : Switch  Criteria=u2 ~= 0  Threshold=2
  Out1 : Outport
  wires:
  EtherCAT PDO Receive9/1 -> Data Type Conversion14/1
  Data Type Conversion14/1 -> MATLAB Function/2(old), Display10/1
  MATLAB Function/1(y) -> Memory/1
  In1/1 -> Switch1/3
  Memory/1 -> Switch1/2, MATLAB Function/1(now)
  Constant/1 -> Switch1/1
  Switch1/1 -> Out1/1

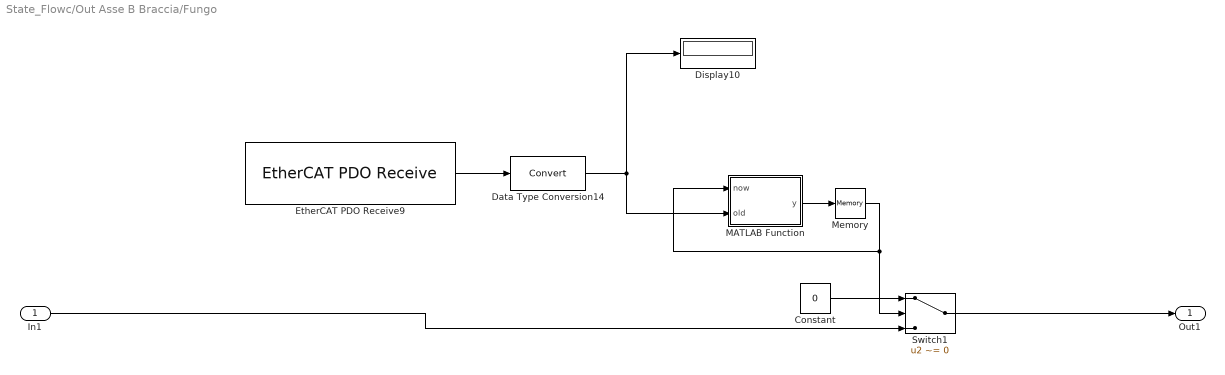
== system State_Flowc/Out Asse B Braccia/Fungo ==
  In1 : Inport
  Constant : Constant  Value=0
  Data Type Conversion14 : DataTypeConversion
  Display10 : Display
  EtherCAT PDO Receive9 : xpcethercatlib/EtherCAT PDO Receive  Priority=2  sig_name=Beckoff.Channel 1.Input  sig_offset=0  sig_type=boolean  type_size=1  sig_dim=1  device_id=0  sample_time=0.001000
      settings: SourceProductName=Simulink Real-Time  SourceProductBaseCode=XP
  MATLAB Function : MATLAB Function  TreatAsAtomicUnit=on
  Memory : Memory
  Switch1 : Switch  Criteria=u2 ~= 0  Threshold=2
  Out1 : Outport
  wires:
  EtherCAT PDO Receive9/1 -> Data Type Conversion14/1
  Data Type Conversion14/1 -> MATLAB Function/2(old), Display10/1
  MATLAB Function/1(y) -> Memory/1
  In1/1 -> Switch1/3
  Memory/1 -> Switch1/2, MATLAB Function/1(now)
  Constant/1 -> Switch1/1
  Switch1/1 -> Out1/1

== system State_Flowc/Out asse A Vite/Fungo ==
  In1 : Inport
  Constant : Constant  Value=0
  Data Type Conversion14 : DataTypeConversion
  Display10 : Display
  EtherCAT PDO Receive9 : xpcethercatlib/EtherCAT PDO Receive  Priority=2  sig_name=Beckoff.Channel 1.Input  sig_offset=0  sig_type=boolean  type_size=1  sig_dim=1  device_id=0  sample_time=0.001000
      settings: SourceProductName=Simulink Real-Time  SourceProductBaseCode=XP
  MATLAB Function : MATLAB Function  TreatAsAtomicUnit=on
  Memory : Memory
  Switch1 : Switch  Criteria=u2 ~= 0  Threshold=2
  Out1 : Outport
  wires:
  EtherCAT PDO Receive9/1 -> Data Type Conversion14/1
  Data Type Conversion14/1 -> MATLAB Function/2(old), Display10/1
  MATLAB Function/1(y) -> Memory/1
  In1/1 -> Switch1/3
  Memory/1 -> Switch1/2, MATLAB Function/1(now)
  Constant/1 -> Switch1/1
  Switch1/1 -> Out1/1

== system State_Flowc/Out asse B Vite/Fungo ==
  In1 : Inport
  Constant : Constant  Value=0
  Data Type Conversion14 : DataTypeConversion
  Display10 : Display
  EtherCAT PDO Receive9 : xpcethercatlib/EtherCAT PDO Receive  Priority=2  sig_name=Beckoff.Channel 1.Input  sig_offset=0  sig_type=boolean  type_size=1  sig_dim=1  device_id=0  sample_time=0.001000
      settings: SourceProductName=Simulink Real-Time  SourceProductBaseCode=XP
  MATLAB Function : MATLAB Function  TreatAsAtomicUnit=on
  Memory : Memory
  Switch1 : Switch  Criteria=u2 ~= 0  Threshold=2
  Out1 : Outport
  wires:
  EtherCAT PDO Receive9/1 -> Data Type Conversion14/1
  Data Type Conversion14/1 -> MATLAB Function/2(old), Display10/1
  MATLAB Function/1(y) -> Memory/1
  In1/1 -> Switch1/3
  Memory/1 -> Switch1/2, MATLAB Function/1(now)
  Constant/1 -> Switch1/1
  Switch1/1 -> Out1/1

== system State_Flowc/Sistema Braccia Linea/Velocita vite  ==
  EtherCAT PDO Receive14 : xpcethercatlib/EtherCAT PDO Receive  Priority=2  sig_name=AZ1.Transmit PDO 1.Axis A Actual motor velocity  sig_offset=48  sig_type=int32  type_size=32  sig_dim=1  device_id=0  sample_time=0.001000
      settings: SourceProductName=Simulink Real-Time  SourceProductBaseCode=XP
  EtherCAT PDO Receive15 : xpcethercatlib/EtherCAT PDO Receive  Priority=2  sig_name=AZ1.Transmit PDO 2.Axis B Actual motor velocity  sig_offset=136  sig_type=int32  type_size=32  sig_dim=1  device_id=0  sample_time=0.001000
      settings: SourceProductName=Simulink Real-Time  SourceProductBaseCode=XP
  Vel Asse A conv : MATLAB Function  TreatAsAtomicUnit=on
  Vel Asse B conv : MATLAB Function  TreatAsAtomicUnit=on
  Velocity A : DataTypeConversion
  Velocity B : DataTypeConversion
  Asse A : Outport
  Asse B : Outport  Port=2
  wires:
  EtherCAT PDO Receive15/1 -> Velocity B/1
  EtherCAT PDO Receive14/1 -> Velocity A/1
  Vel Asse A conv/1(vel_A_conv) -> Asse A/1
  Velocity B/1 -> Vel Asse B conv/1(p)
  Vel Asse B conv/1(vel_B_conv) -> Asse B/1
  Velocity A/1 -> Vel Asse A conv/1(vA)

== system State_Flowc/Sistema Vite/Actual A ==
  Pos : Inport
  Offset : Inport  Port=2
  Rif asse B : Inport  Port=3
  Discrete Derivative A : simulink/Discrete/Discrete Derivative  gainval=1.0  ICPrevScaledInput=0.0  OutMin=[]  OutMax=[]  OutDataType=fixdt(1, 16)  OutScaling=2^-10  DoSatur=off
  Display31 : Display
  Posizione attuale Vite A : Subsystem
  Sum : Sum  Inputs=|-+
  A attuale : Outport
  wires:
  Offset/1 -> Sum/1
  Posizione attuale Vite A/1(A Att) -> A attuale/1, Discrete Derivative A/1
  Sum/1 -> Posizione attuale Vite A/1(Comp Vite A)
  Rif asse B/1 -> Posizione attuale Vite A/2("Comp Vite B ")
  Pos/1 -> Sum/2
  Discrete Derivative A/1 -> Display31/1

== system State_Flowc/Sistema Vite/Clock reale ==
  cr : Inport
  offset : Inport  Port=2
  Sum2 : Sum  Inputs=-+|
  Ck : Outport
  wires:
  Sum2/1 -> Ck/1
  offset/1 -> Sum2/1
  cr/1 -> Sum2/2

== system State_Flowc/Sistema Vite/Coppia VIte A finale ==
  Pos : Inport
  Vel : Inport  Port=2
  Gain : Gain  Gain=300*1000/0.36
  Gain6 : Gain  Gain=7.5*1000/0.36
  Sum9 : Sum  Inputs=|++
  Coppia : Outport
  wires:
  Pos/1 -> Gain/1
  Sum9/1 -> Coppia/1
  Gain6/1 -> Sum9/2
  Vel/1 -> Gain6/1
  Gain/1 -> Sum9/1

== system State_Flowc/Sistema Vite/Velocita vite  ==
  EtherCAT PDO Receive14 : xpcethercatlib/EtherCAT PDO Receive  Priority=2  sig_name=AZ2.Transmit PDO 1.Axis A Actual motor velocity  sig_offset=304  sig_type=int32  type_size=32  sig_dim=1  device_id=0  sample_time=0.001000
      settings: SourceProductName=Simulink Real-Time  SourceProductBaseCode=XP
  EtherCAT PDO Receive15 : xpcethercatlib/EtherCAT PDO Receive  Priority=2  sig_name=AZ2.Transmit PDO 2.Axis B Actual motor velocity  sig_offset=392  sig_type=int32  type_size=32  sig_dim=1  device_id=0  sample_time=0.001000
      settings: SourceProductName=Simulink Real-Time  SourceProductBaseCode=XP
  Vel Asse A conv : MATLAB Function  TreatAsAtomicUnit=on
  Vel Asse B conv : MATLAB Function  TreatAsAtomicUnit=on
  Velocity A : DataTypeConversion
  Velocity B : DataTypeConversion
  Asse A : Outport
  Asse B : Outport  Port=2
  wires:
  EtherCAT PDO Receive15/1 -> Velocity B/1
  EtherCAT PDO Receive14/1 -> Velocity A/1
  Vel Asse A conv/1(vel_A_conv) -> Asse A/1
  Velocity B/1 -> Vel Asse B conv/1(p), Vel Asse A conv/2(vB)
  Vel Asse B conv/1(vel_B_conv) -> Asse B/1
  Velocity A/1 -> Vel Asse A conv/1(vA)

== system State_Flowc/State flow robot/Mov1/Clock reale ==
  cr : Inport
  offset : Inport  Port=2
  Sum2 : Sum  Inputs=-+|
  Ck : Outport
  wires:
  Sum2/1 -> Ck/1
  offset/1 -> Sum2/1
  cr/1 -> Sum2/2

== system State_Flowc/Movimento Braccia/Coppie braccia/Velocita vite  ==
  EtherCAT PDO Receive14 : xpcethercatlib/EtherCAT PDO Receive  Priority=2  sig_name=AZ1.Transmit PDO 2.Axis B Actual motor velocity  sig_offset=136  sig_type=int32  type_size=32  sig_dim=1  device_id=0  sample_time=0.001
      settings: SourceProductName=Simulink Real-Time  SourceProductBaseCode=XP
  EtherCAT PDO Receive15 : xpcethercatlib/EtherCAT PDO Receive  Priority=2  sig_name=AZ1.Transmit PDO 1.Axis A Actual motor velocity  sig_offset=48  sig_type=int32  type_size=32  sig_dim=1  device_id=0  sample_time=0.001
      settings: SourceProductName=Simulink Real-Time  SourceProductBaseCode=XP
  Vel Asse A conv : MATLAB Function  TreatAsAtomicUnit=on
  Vel Asse B conv : MATLAB Function  TreatAsAtomicUnit=on
  Velocity A : DataTypeConversion
  Velocity B : DataTypeConversion
  Asse B : Outport
  Asse A : Outport  Port=2
  wires:
  EtherCAT PDO Receive15/1 -> Velocity A/1
  EtherCAT PDO Receive14/1 -> Velocity B/1
  Vel Asse B conv/1(vel_B_conv) -> Asse B/1
  Velocity A/1 -> Vel Asse A conv/1(vA)
  Vel Asse A conv/1(vel_A_conv) -> Asse A/1
  Velocity B/1 -> Vel Asse B conv/1(vB)

== system State_Flowc/Sistema Vite/Actual A/Posizione attuale Vite A ==
  Comp Vite A : Inport
  "Comp Vite B " : Inport  Port=2
  Asse A conv : MATLAB Function  TreatAsAtomicUnit=on
  Asse B conv v : MATLAB Function  TreatAsAtomicUnit=on
  Sum5 : Sum
  A Att : Outport
  wires:
  Asse A conv/1(pos_A_conv) -> Sum5/1
  Asse B conv v/1(pos_B_conv_v) -> Sum5/2
  Comp Vite A/1 -> Asse A conv/1(p)
  Sum5/1 -> A Att/1
  "Comp Vite B "/1 -> Asse B conv v/1(p)

== matlab function State_Flowc/Movimento Braccia/Cinematica Inversa iniziale ==
  data: x0old input; y0old input; theta1_0 input; theta2_0 input; time input; x0 output; y0 output
function [x0, y0] = CinInvIniziale(x0old, y0old, theta1_0, theta2_0, time)

if time == 0 

d = 0.09; 
l = 0.25;

A = l^2*(sin(theta2_0)-sin(theta1_0))^2 + (-2*d -l*(cos(theta2_0)-cos(theta1_0)))^2;
B = -2*l^2*d*(sin(theta2_0)-sin(theta1_0))*(cos(theta2_0)+cos(theta1_0)) + ...
    l*(sin(theta2_0)-sin(theta1_0))*(-2*d -l*(cos(theta2_0)-cos(theta1_0)))*(-2*d -2*l*cos(theta2_0)) - ...
    2*l*sin(theta2_0)*(-2*d -l*(cos(theta2_0)-cos(theta1_0)))^2;
C = l^2*d^2*(cos(theta2_0)+cos(theta1_0))^2 -l*d*(cos(theta2_0)+cos(theta1_0))*(-2*d -l*(cos(theta2_0)-cos(theta1_0)))*(-2*d -2*l*cos(theta2_0)) + ...
    (d^2 + 2*d*l*cos(theta2_0))*(-2*d - l*(cos(theta2_0)-cos(theta1_0)))^2;

% Posizione Y end-effector
y0 = (-B + sqrt(B^2 - 4*A*C))/(2*A);
% Posizione X end-effector
x0 = (y0*l*(sin(theta2_0)-sin(theta1_0)) - l*d*(cos(theta2_0)+cos(theta1_0)))/(-2*d -l*(cos(theta2_0)-cos(theta1_0)));
else 
    x0 = x0old;
    y0 = y0old;
end
